simulink model "exampleModell"  (R2018b)
settings: Solver=VariableStepAuto  StartTime=0.0  StopTime=1  RelTol=1e-3
StartFcn:
  | % Set up the arguments that will go into the gain block event callback listener
  | blk1 = 'exampleModell/Out1';
  | blk2 = 'exampleModell/Out2';
  | 
  | 
  | event = 'PostOutputs';
  | listener = @updateApp;
  | 
  | % Create the listener
  | h1 = add_exec_event_listener(blk1, event, listener);
  | h2 = add_exec_event_listener(blk2, event, listener);
undefined symbols (not defined in the file): constantVal, gainVal
settings Model: Creator=ulzymfv  LastModifiedBy=ulzymfv

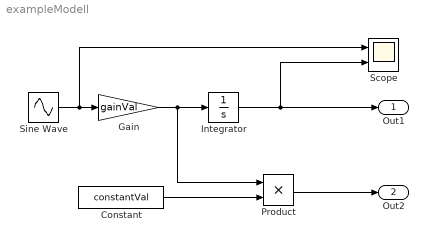
== system exampleModell ==
  Constant : Constant  Value=constantVal
  Gain : Gain  Gain=gainVal
  Integrator : Integrator
  Product : Product
  Scope : Scope  NumInputPorts=2
  Sine Wave : Sin  SampleTime=0
  Out1 : Outport
  Out2 : Outport  Port=2
  wires:
  Sine Wave/1 -> Scope/1, Gain/1
  Gain/1 -> Product/1, Integrator/1
  Integrator/1 -> Scope/2, Out1/1
  Constant/1 -> Product/2
  Product/1 -> Out2/1
